simulink model "Suspension_Shaker_Model_Assignment"  (R2022b)
settings: Solver=FixedStepAuto  StartTime=0.0  StopTime=100  FixedStep=0.005  RelTol=1e-3
values from neighbouring files (symbols this model uses):
  A = 1.25    [Suspension_Shaker_Model_Parameters.m]
  a = 1.80    (= 1.8)    [Suspension_Shaker_Model_Parameters.m]
  b = L-a    (= 1.7)    [Suspension_Shaker_Model_Parameters.m]
  cdf = 1400    [Suspension_Shaker_Model_Parameters.m]
  cdr = 1800    [Suspension_Shaker_Model_Parameters.m]
  cz = 1    [Suspension_Shaker_Model_Parameters.m]
  F0f = ms_front*g    (= 1870.20642857)    [Suspension_Shaker_Model_Parameters.m]
  F0r = ms_rear*g    (= 1980.21857143)    [Suspension_Shaker_Model_Parameters.m]
  g = 9.81    [Suspension_Shaker_Model_Parameters.m]
  h = 0.2    [Suspension_Shaker_Model_Parameters.m]
  hrc = 0.05    [Suspension_Shaker_Model_Parameters.m]
  hrcf = 0.04    [Suspension_Shaker_Model_Parameters.m]
  hrcr = 0.06    [Suspension_Shaker_Model_Parameters.m]
  Ixx = 300    [Suspension_Shaker_Model_Parameters.m]
  Iyy = 1350    [Suspension_Shaker_Model_Parameters.m]
  karbf = 5000    [Suspension_Shaker_Model_Parameters.m]
  karbr = 1000    [Suspension_Shaker_Model_Parameters.m]
  ksf = 67500    [Suspension_Shaker_Model_Parameters.m]
  ksr = 100000    [Suspension_Shaker_Model_Parameters.m]
  ktyre = 400000    [Suspension_Shaker_Model_Parameters.m]
  L = 3.5    [Suspension_Shaker_Model_Parameters.m]
  ms = m - (2*musr) - (2*musf)    (= 785)    [Suspension_Shaker_Model_Parameters.m]
  musf = 15    [Suspension_Shaker_Model_Parameters.m]
  musr = 17.50    (= 17.5)    [Suspension_Shaker_Model_Parameters.m]
  r = 0.375    [Suspension_Shaker_Model_Parameters.m]
  rho = 1.225    [Suspension_Shaker_Model_Parameters.m]
  tr = 1.85    [Suspension_Shaker_Model_Parameters.m]
  z0ft = (ms_front + musf) * (g/ktyre)    (= 0.00504339107143)    [Suspension_Shaker_Model_Parameters.m]
  z0rt = (ms_rear + musr) * (g/ktyre)    (= 0.00537973392857)    [Suspension_Shaker_Model_Parameters.m]
libraries: simulink_extras x4, simulink x1
settings Model: Creator=webstert  LastModifiedBy=webstert

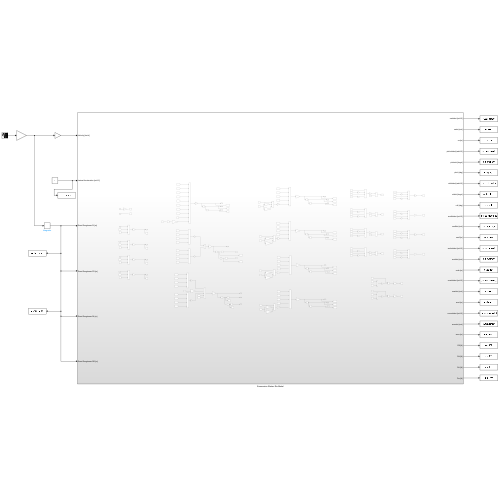
[thumbnail: Simulink's stored preview of the top-level diagram]
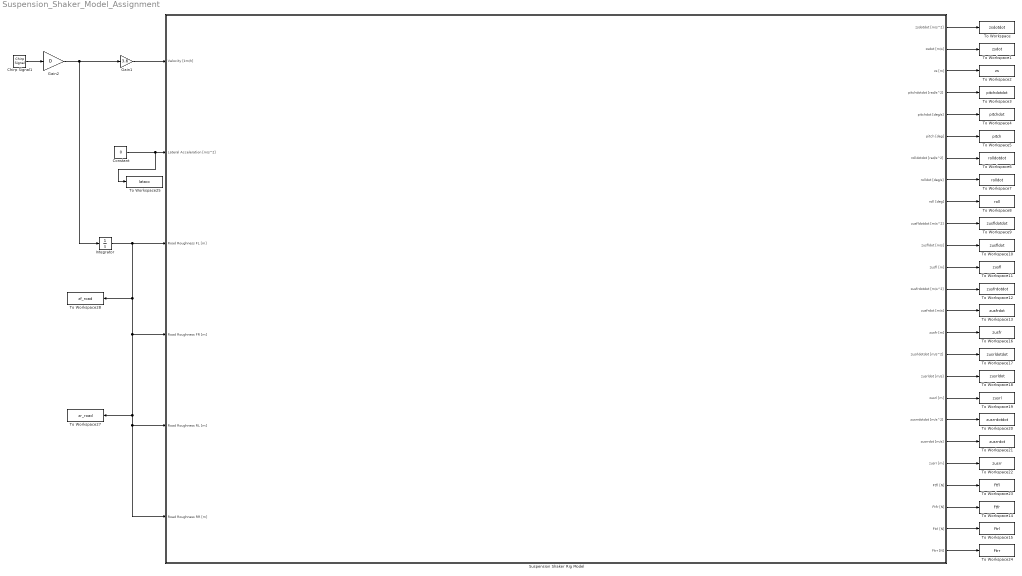
== system Suspension_Shaker_Model_Assignment ==
  Chirp Signal1 : simulink/Sources/Chirp Signal  f1=0.1  T=100  f2=50
  Constant : Constant  Value=0
  Gain1 : Gain  Gain=3.6
  Gain2 : Gain  Gain=0
  Integrator : Integrator
  Suspension Shaker Rig Model : Subsystem
  To Workspace : ToWorkspace  VariableName=zsdotdot  SaveFormat=Timeseries  SampleTime=-1
  To Workspace1 : ToWorkspace  VariableName=zsdot  SaveFormat=Timeseries  SampleTime=-1
  To Workspace10 : ToWorkspace  VariableName=zusfldot  SaveFormat=Timeseries  SampleTime=-1
  To Workspace11 : ToWorkspace  VariableName=zusfl  SaveFormat=Timeseries  SampleTime=-1
  To Workspace12 : ToWorkspace  VariableName=zusfrdotdot  SaveFormat=Timeseries  SampleTime=-1
  To Workspace13 : ToWorkspace  VariableName=zusfrdot  SaveFormat=Timeseries  SampleTime=-1
  To Workspace14 : ToWorkspace  VariableName=Ftfr  SaveFormat=Timeseries  SampleTime=-1
  To Workspace15 : ToWorkspace  VariableName=Ftrl  SaveFormat=Timeseries  SampleTime=-1
  To Workspace16 : ToWorkspace  VariableName=zusfr  SaveFormat=Timeseries  SampleTime=-1
  To Workspace17 : ToWorkspace  VariableName=zusrldotdot  SaveFormat=Timeseries  SampleTime=-1
  To Workspace18 : ToWorkspace  VariableName=zusrldot  SaveFormat=Timeseries  SampleTime=-1
  To Workspace19 : ToWorkspace  VariableName=zusrl  SaveFormat=Timeseries  SampleTime=-1
  To Workspace2 : ToWorkspace  VariableName=zs  SaveFormat=Timeseries  SampleTime=-1
  To Workspace20 : ToWorkspace  VariableName=zusrrdotdot  SaveFormat=Timeseries  SampleTime=-1
  To Workspace21 : ToWorkspace  VariableName=zusrrdot  SaveFormat=Timeseries  SampleTime=-1
  To Workspace22 : ToWorkspace  VariableName=zusrr  SaveFormat=Timeseries  SampleTime=-1
  To Workspace23 : ToWorkspace  VariableName=Ftfl  SaveFormat=Timeseries  SampleTime=-1
  To Workspace24 : ToWorkspace  VariableName=Ftrr  SaveFormat=Timeseries  SampleTime=-1
  To Workspace25 : ToWorkspace  VariableName=latacc  SaveFormat=Timeseries  SampleTime=-1
  To Workspace27 : ToWorkspace  VariableName=zr_road  SaveFormat=Timeseries  SampleTime=-1
  To Workspace28 : ToWorkspace  VariableName=zf_road  SaveFormat=Timeseries  SampleTime=-1
  To Workspace3 : ToWorkspace  VariableName=pitchdotdot  SaveFormat=Timeseries  SampleTime=-1
  To Workspace4 : ToWorkspace  VariableName=pitchdot  SaveFormat=Timeseries  SampleTime=-1
  To Workspace5 : ToWorkspace  VariableName=pitch  SaveFormat=Timeseries  SampleTime=-1
  To Workspace6 : ToWorkspace  VariableName=rolldotdot  SaveFormat=Timeseries  SampleTime=-1
  To Workspace7 : ToWorkspace  VariableName=rolldot  SaveFormat=Timeseries  SampleTime=-1
  To Workspace8 : ToWorkspace  VariableName=roll  SaveFormat=Timeseries  SampleTime=-1
  To Workspace9 : ToWorkspace  VariableName=zusfldotdot  SaveFormat=Timeseries  SampleTime=-1
  wires:
  Gain2/1 -> Integrator/1, Gain1/1
  Constant/1 -> To Workspace25/1, Suspension Shaker Rig Model/2(Lateral Acceleration [m/s^2])
  Suspension Shaker Rig Model/1(zsdotdot [m/s^2]) -> To Workspace/1
  Suspension Shaker Rig Model/2(zsdot [m/s]) -> To Workspace1/1
  Suspension Shaker Rig Model/3(zs [m]) -> To Workspace2/1
  Suspension Shaker Rig Model/5(pitchdot [deg/s]) -> To Workspace4/1
  Suspension Shaker Rig Model/6(pitch [deg]) -> To Workspace5/1
  Suspension Shaker Rig Model/4(pitchdotdot [rad/s^2]) -> To Workspace3/1
  Suspension Shaker Rig Model/8(rolldot [deg/s]) -> To Workspace7/1
  Suspension Shaker Rig Model/11(zusfldot [m/s]) -> To Workspace10/1
  Suspension Shaker Rig Model/9(roll [deg]) -> To Workspace8/1
  Suspension Shaker Rig Model/7(rolldotdot [rad/s^2]) -> To Workspace6/1
  Suspension Shaker Rig Model/12(zusfl [m]) -> To Workspace11/1
  Suspension Shaker Rig Model/10(zusfldotdot [m/s^2]) -> To Workspace9/1
  Suspension Shaker Rig Model/22(Ftfl [N]) -> To Workspace23/1
  Suspension Shaker Rig Model/21(zusrr [m]) -> To Workspace22/1
  Suspension Shaker Rig Model/19(zusrrdotdot [m/s^2]) -> To Workspace20/1
  Suspension Shaker Rig Model/20(zusrrdot [m/s]) -> To Workspace21/1
  Suspension Shaker Rig Model/24(Ftrl [N]) -> To Workspace15/1
  Suspension Shaker Rig Model/14(zusfrdot [m/s]) -> To Workspace13/1
  Suspension Shaker Rig Model/23(Ftfr [N]) -> To Workspace14/1
  Suspension Shaker Rig Model/17(zusrldot [m/s]) -> To Workspace18/1
  Suspension Shaker Rig Model/15(zusfr [m]) -> To Workspace16/1
  Suspension Shaker Rig Model/13(zusfrdotdot [m/s^2]) -> To Workspace12/1
  Suspension Shaker Rig Model/16(zusrldotdot [m/s^2]) -> To Workspace17/1
  Suspension Shaker Rig Model/18(zusrl [m]) -> To Workspace19/1
  Suspension Shaker Rig Model/25(Ftrr [N]) -> To Workspace24/1
  Chirp Signal1/1 -> Gain2/1
  Integrator/1 -> To Workspace28/1, Suspension Shaker Rig Model/6(Road Roughness RR [m]), Suspension Shaker Rig Model/5(Road Roughness RL [m]), To Workspace27/1, Suspension Shaker Rig Model/4(Road Roughness FR [m]), Suspension Shaker Rig Model/3(Road Roughness FL [m])
  Gain1/1 -> Suspension Shaker Rig Model/1(Velocity [km/h])

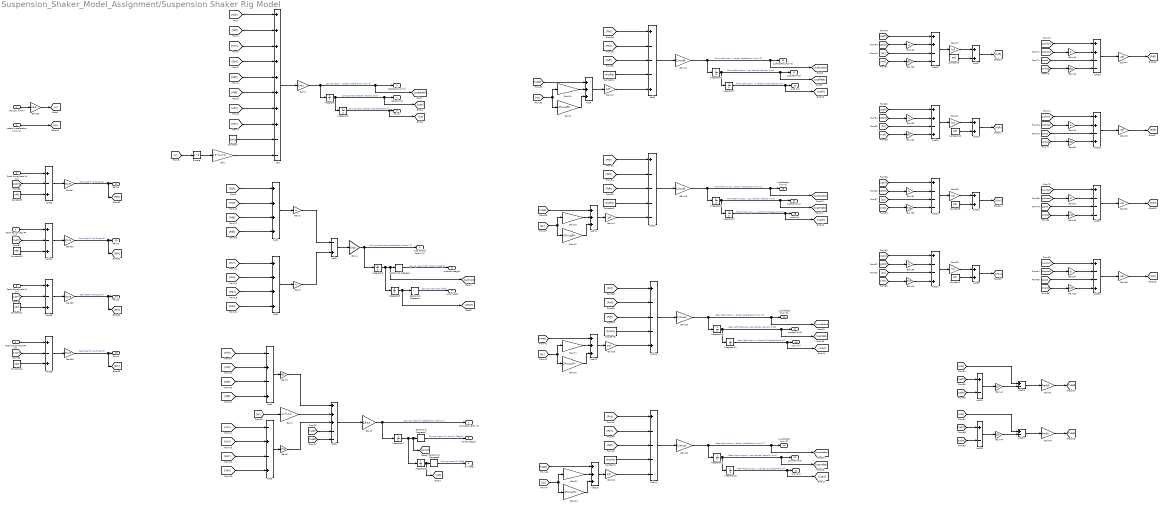
== system Suspension_Shaker_Model_Assignment/Suspension Shaker Rig Model ==
  Velocity [km/h] : Inport
  Lateral Acceleration [m/s^2] : Inport  Port=2
  Road Roughness FL [m] : Inport  Port=3
  Road Roughness FR [m] : Inport  Port=4
  Road Roughness RL [m] : Inport  Port=5
  Road Roughness RR [m] : Inport  Port=6
  Add : Sum  Inputs=++++++++--
  Add1 : Sum  Inputs=++++
  Add10 : Sum  Inputs=+----
  Add{9,11,13,15} (4 alike) : Sum  Inputs=+++
  Add12 : Sum  Inputs=+---+
  Add14 : Sum  Inputs=+----
  Add16 : Sum  Inputs=++--
  Add{17,19,21,23} (4 alike) : Sum
  Add18 : Sum  Inputs=++-+
  Add2 : Sum  Inputs=++++
  Add20 : Sum  Inputs=+---
  Add22 : Sum  Inputs=+--+
  Add{24..27} (4 alike) : Sum  Inputs=+-
  Add28 : Sum  Inputs=++--
  Add29 : Sum  Inputs=++-+
  Add3 : Sum  Inputs=-+
  Add30 : Sum  Inputs=+---
  Add31 : Sum  Inputs=+--+
  Add{32,34,36,38} (4 alike) : Sum  Inputs=+-+
  Add4 : Sum  Inputs=-+-+
  Add5 : Sum  Inputs=-+-+
  Add6 : Sum  Inputs=+++--
  Add8 : Sum  Inputs=+---+
  Constant : Constant  Value=ms*g
  Constant1 : Constant  Value=musf*g
  Constant10 : Constant  Value=z0ft
  Constant11 : Constant  Value=z0rt
  Constant12 : Constant  Value=z0rt
  Constant13 : Constant  Value=F0f
  Constant2 : Constant  Value=musf*g
  Constant3 : Constant  Value=musr*g
  Constant4 : Constant  Value=musr*g
  Constant5 : Constant  Value=F0r
  Constant6 : Constant  Value=F0f
  Constant7 : Constant  Value=F0r
  Constant9 : Constant  Value=z0ft
  Gain : Gain  Gain=0.5*rho*A*cz
  Gain1 : Gain  Gain=1/ms
  Gain10 : Gain  Gain=ms*hrcf*(b/L)
  Gain11 : Gain  Gain=1/tf
  Gain12 : Gain  Gain=1/musf
  Gain13 : Gain  Gain=ms*hrcf*(b/L)
  Gain14 : Gain  Gain=1/tf
  Gain15 : Gain  Gain=1/musf
  Gain16 : Gain  Gain=2*musf*r
  Gain17 : Gain  Gain=ms*hrcr*(a/L)
  Gain18 : Gain  Gain=1/tr
  Gain19 : Gain  Gain=1/musr
  Gain{2,26,30,45..46} (5 alike) : Gain  Gain=a
  Gain20 : Gain  Gain=2*musr*r
  Gain21 : Gain  Gain=ms*hrcr*(a/L)
  Gain22 : Gain  Gain=1/tr
  Gain23 : Gain  Gain=1/musr
  Gain24 : Gain  Gain=2*musr*r
  Gain25 : Gain  Gain=1/3.6
  Gain27 : Gain  Gain=ksf
  Gain{5,28,32,48,50} (5 alike) : Gain  Gain=tf/2
  Gain{3,34,38,51,54} (5 alike) : Gain  Gain=b
  Gain31 : Gain  Gain=ksf
  Gain35 : Gain  Gain=ksr
  Gain{6,36,40,53,56} (5 alike) : Gain  Gain=tr/2
  Gain39 : Gain  Gain=ksr
  Gain4 : Gain  Gain=1/Iyy
  Gain41 : Gain  Gain=karbf
  Gain42 : Gain  Gain=1/tf
  Gain43 : Gain  Gain=karbr
  Gain44 : Gain  Gain=1/tr
  Gain47 : Gain  Gain=cdf
  Gain49 : Gain  Gain=cdf
  Gain52 : Gain  Gain=cdr
  Gain55 : Gain  Gain=cdr
  Gain{57,60,63,66} (4 alike) : Gain  Gain=ktyre
  Gain7 : Gain  Gain=ms*(h-hrc)
  Gain8 : Gain  Gain=1/Ixx
  Gain9 : Gain  Gain=2*musf*r
  Integrator{,1..13} (14 alike) : Integrator
  Radians to Degrees{,1..3} (4 alike) : simulink_extras/Transformations/Radians to Degrees
  Square : Math  Operator=square
  zsdotdot [m/s^2] : Outport
  zsdot [m/s] : Outport  Port=2
  zs [m] : Outport  Port=3
  pitchdotdot [rad/s^2] : Outport  Port=4
  pitchdot [deg/s] : Outport  Port=5
  pitch [deg] : Outport  Port=6
  rolldotdot [rad/s^2] : Outport  Port=7
  rolldot [deg/s] : Outport  Port=8
  roll [deg] : Outport  Port=9
  zusfldotdot [m/s^2] : Outport  Port=10
  zusfldot [m/s] : Outport  Port=11
  zusfl [m] : Outport  Port=12
  zusfrdotdot [m/s^2] : Outport  Port=13
  zusfrdot [m/s] : Outport  Port=14
  zusfr [m] : Outport  Port=15
  zusrldotdot [m/s^2] : Outport  Port=16
  zusrldot [m/s] : Outport  Port=17
  zusrl [m] : Outport  Port=18
  zusrrdotdot [m/s^2] : Outport  Port=19
  zusrrdot [m/s] : Outport  Port=20
  zusrr [m] : Outport  Port=21
  Ftfl [N] : Outport  Port=22
  Ftfr [N] : Outport  Port=23
  Ftrl [N] : Outport  Port=24
  Ftrr [N] : Outport  Port=25
  wires:
  Add/1 -> Gain1/1
  Square/1 -> Gain/1
  [Fdfr] -> Add/5
  [Fsrl] -> Add/4
  [Fdrr] -> Add/7
  [Fdfl] -> Add/6
  [Fsfl] -> Add/2
  [Fsrr] -> Add/3
  Constant/1 -> Add/9
  [Fsfr] -> Add/1
  [V] -> Square/1
  [Fdrl] -> Add/8
  Gain/1 -> Add/10
  Gain1/1 -> Integrator/1, [zsdotdot], zsdotdot [m/s^2]/1  "Sprung Mass Vertical Acceleration [m/s^2]"
  Velocity [km/h]/1 -> Gain25/1
  Integrator1/1 -> [zs], zs [m]/1  "Sprung Mass Vertical Displacement [m]"
  Integrator/1 -> Integrator1/1, [zsdot], zsdot [m/s]/1  "Sprung Mass Vertical Velocity [m/s]"
  [Fsfr] -> Add1/1
  [Fsfl] -> Add1/2
  [Fdrl] -> Add2/4
  [Fdrr] -> Add2/3
  [Fdfr] -> Add1/3
  [Fdfl] -> Add1/4
  [Fsrr] -> Add2/1
  [Fsrl] -> Add2/2
  Add1/1 -> Gain2/1
  Add2/1 -> Gain3/1
  Gain2/1 -> Add3/1
  Gain3/1 -> Add3/2
  Add3/1 -> Gain4/1
  Gain4/1 -> Integrator2/1, pitchdotdot [rad/s^2]/1  "Sprung mass pitch acceleration [rad/s^2]"
  Integrator2/1 -> Integrator3/1, [pitchdot], Radians to Degrees/1
  Integrator3/1 -> [pitch], Radians to Degrees1/1
  Radians to Degrees/1 -> pitchdot [deg/s]/1  "Sprung mass pitch velocity [deg/s]"
  Radians to Degrees1/1 -> pitch [deg]/1  "Sprung mass ptich [deg]"
  [Fdrl] -> Add5/4
  [Fsrr] -> Add5/1
  [Fsrl] -> Add5/2
  [Fdfl] -> Add4/4
  [Fdfr] -> Add4/3
  [Fsfl] -> Add4/2
  [Fdrr] -> Add5/3
  [Fsfr] -> Add4/1
  Gain5/1 -> Add6/1
  Gain6/1 -> Add6/3
  Add4/1 -> Gain5/1
  Add5/1 -> Gain6/1
  [ay] -> Gain7/1
  Gain7/1 -> Add6/2
  [TARBf] -> Add6/5
  [TARBr] -> Add6/4
  Add6/1 -> Gain8/1
  Gain8/1 -> Integrator4/1, rolldotdot [rad/s^2]/1  "Sprung mass roll acceleration [rad/s^2]"
  Integrator5/1 -> [roll], Radians to Degrees3/1
  Integrator4/1 -> Integrator5/1, [rolldot], Radians to Degrees2/1
  Radians to Degrees2/1 -> rolldot [deg/s]/1  "Sprung mass roll velocity [deg/s]"
  Radians to Degrees3/1 -> roll [deg]/1  "Sprung mass roll [deg]"
  [Fsfl] -> Add8/2
  [Fdfl] -> Add8/3
  [Ftfl] -> Add8/1
  Integrator7/1 -> [zusfl], zusfl [m]/1  "Front Left Unsprung Mass Vertical Displacement [m]"
  Integrator6/1 -> Integrator7/1, [zusfldot], zusfldot [m/s]/1  "Front Left Unsprung Mass Vertical Velocity [m/s]"
  Constant1/1 -> Add8/4
  Add8/1 -> Gain12/1
  Gain12/1 -> Integrator6/1, [zusfldotdot], zusfldotdot [m/s^2]/1  "Front Left Unsprung Mass Vertical Acceleration [m/s^2]"
  [ay] -> Gain10/1, Gain9/1
  [TARBf] -> Add9/1
  Gain10/1 -> Add9/2
  Gain9/1 -> Add9/3
  Add9/1 -> Gain11/1
  Gain11/1 -> Add8/5
  Gain16/1 -> Add11/3
  [TARBf] -> Add11/1
  Gain15/1 -> Integrator8/1, [zusfrdotdot], zusfrdotdot [m/s^2]/1  "Front Right Unsprung Mass Vertical Acceleration [m/s^2]"
  Add11/1 -> Gain14/1
  Constant2/1 -> Add10/4
  Gain13/1 -> Add11/2
  Gain14/1 -> Add10/5
  Integrator9/1 -> [zusfr], zusfr [m]/1  "Front Right Unsprung Mass Vertical Displacement [m]"
  [Fsfr] -> Add10/2
  [Ftfr] -> Add10/1
  Add10/1 -> Gain15/1
  Integrator8/1 -> Integrator9/1, [zusfrdot], zusfrdot [m/s]/1  "Front Right Unsprung Mass Vertical Velocity [m/s]"
  [Fdfr] -> Add10/3
  [ay] -> Gain13/1, Gain16/1
  Gain20/1 -> Add13/3
  [TARBr] -> Add13/1
  Gain19/1 -> Integrator10/1, [zusrldotdot], zusrldotdot [m/s^2]/1  "Rear Left Unsprung Mass Vertical Acceleration [m/s^2]"
  Add13/1 -> Gain18/1
  Constant3/1 -> Add12/4
  Gain17/1 -> Add13/2
  Gain18/1 -> Add12/5
  Integrator11/1 -> [zusrl], zusrl [m]/1  "Rear Left Unsprung Mass Vertical Displacement [m]"
  [Fsrl] -> Add12/2
  [Ftrl] -> Add12/1
  Add12/1 -> Gain19/1
  Integrator10/1 -> Integrator11/1, [zusrldot], zusrldot [m/s]/1  "Rear Left Unsprung Mass Vertical Velocity [m/s]"
  [Fdrl] -> Add12/3
  [ay] -> Gain17/1, Gain20/1
  Integrator12/1 -> Integrator13/1, [zusrrdot], zusrrdot [m/s]/1  "Rear Right Unsprung Mass Vertical Velocity [m/s]"
  [Fdrr] -> Add14/3
  Constant4/1 -> Add14/4
  [Ftrr] -> Add14/1
  Add14/1 -> Gain23/1
  [Fsrr] -> Add14/2
  Integrator13/1 -> [zusrr], zusrr [m]/1  "Rear Right Unsprung Mass Vertical Displacement [m]"
  [ay] -> Gain21/1, Gain24/1
  Gain24/1 -> Add15/3
  Gain21/1 -> Add15/2
  Gain23/1 -> Integrator12/1, [zusrrdotdot], zusrrdotdot [m/s^2]/1  "Rear Right Unsprung Mass Vertical Acceleration [m/s^2]"
  [TARBr] -> Add15/1
  Add15/1 -> Gain22/1
  Gain22/1 -> Add14/5
  Constant6/1 -> Add17/2
  Gain27/1 -> Add17/1
  [zusfl] -> Add16/1
  [pitch] -> Gain26/1
  [zs] -> Add16/3
  [roll] -> Gain28/1
  Gain28/1 -> Add16/4
  Gain26/1 -> Add16/2
  Add16/1 -> Gain27/1
  Add17/1 -> [Fsfl]
  [roll] -> Gain32/1
  Gain30/1 -> Add18/2
  Gain32/1 -> Add18/4
  Gain31/1 -> Add19/1
  [zusfr] -> Add18/1
  [zs] -> Add18/3
  Add19/1 -> [Fsfr]
  Add18/1 -> Gain31/1
  [pitch] -> Gain30/1
  [roll] -> Gain36/1
  Gain34/1 -> Add20/2
  Gain36/1 -> Add20/4
  Gain35/1 -> Add21/1
  [zusrl] -> Add20/1
  [zs] -> Add20/3
  Add21/1 -> [Fsrl]
  Add20/1 -> Gain35/1
  [pitch] -> Gain34/1
  [pitch] -> Gain38/1
  [zusrr] -> Add22/1
  [zs] -> Add22/3
  Gain40/1 -> Add22/4
  [roll] -> Gain40/1
  Add22/1 -> Gain39/1
  Gain39/1 -> Add23/1
  Gain38/1 -> Add22/2
  Add23/1 -> [Fsrr]
  [zusfr] -> Add24/2
  [zusfl] -> Add24/1
  Add24/1 -> Gain42/1
  [roll] -> Add25/1
  Gain42/1 -> Add25/2
  Add25/1 -> Gain41/1
  Gain41/1 -> [TARBf]
  Add27/1 -> Gain43/1
  Add26/1 -> Gain44/1
  [zusrl] -> Add26/1
  Gain44/1 -> Add27/2
  [zusrr] -> Add26/2
  [roll] -> Add27/1
  Gain43/1 -> [TARBr]
  [rolldot] -> Gain48/1
  Gain46/1 -> Add28/2
  Gain48/1 -> Add28/4
  [zusfldot] -> Add28/1
  [zsdot] -> Add28/3
  Gain47/1 -> [Fdfl]
  Add28/1 -> Gain47/1
  [pitchdot] -> Gain46/1
  [pitchdot] -> Gain45/1
  [zusfrdot] -> Add29/1
  [rolldot] -> Gain50/1
  [zsdot] -> Add29/3
  Gain50/1 -> Add29/4
  Gain45/1 -> Add29/2
  Gain49/1 -> [Fdfr]
  Add29/1 -> Gain49/1
  [pitchdot] -> Gain51/1
  [zusrldot] -> Add30/1
  [rolldot] -> Gain53/1
  [zsdot] -> Add30/3
  Gain53/1 -> Add30/4
  Gain51/1 -> Add30/2
  Gain52/1 -> [Fdrl]
  Add30/1 -> Gain52/1
  [zusrrdot] -> Add31/1
  [rolldot] -> Gain56/1
  Add31/1 -> Gain55/1
  Gain55/1 -> [Fdrr]
  Gain56/1 -> Add31/4
  [pitchdot] -> Gain54/1
  Gain54/1 -> Add31/2
  [zsdot] -> Add31/3
  Road Roughness FL [m]/1 -> Add32/1
  [zusfl] -> Add32/2
  Add32/1 -> Gain57/1
  Gain57/1 -> [Ftfl], Ftfl [N]/1  "Front Left Tyre Force [N]"
  Constant9/1 -> Add32/3
  Constant10/1 -> Add34/3
  Road Roughness FR [m]/1 -> Add34/1
  Add34/1 -> Gain60/1
  Gain60/1 -> [Ftfr], Ftfr [N]/1  "Front Right Tyre Force [N]"
  [zusfr] -> Add34/2
  Constant11/1 -> Add36/3
  Road Roughness RL [m]/1 -> Add36/1
  Add36/1 -> Gain63/1
  Gain63/1 -> [Ftrl], Ftrl [N]/1  "Rear Left Tyre Force [N]"
  [zusrl] -> Add36/2
  [zusrr] -> Add38/2
  Gain66/1 -> [Ftrr], Ftrr [N]/1  "Rear Right Tyre Force [N]"
  Add38/1 -> Gain66/1
  Constant12/1 -> Add38/3
  Road Roughness RR [m]/1 -> Add38/1
  Lateral Acceleration [m/s^2]/1 -> [ay]
  Constant13/1 -> Add19/2
  Constant5/1 -> Add21/2
  Constant7/1 -> Add23/2
  Gain25/1 -> [V]
